simulink model "train_network"  (R2019a)
settings: Solver=VariableStepAuto  StartTime=0.0  StopTime=2400  RelTol=1e-3
values from neighbouring files (symbols this model uses):
  door_opening = [15 15 15 15 15 15 15]    [get_parameters.m]
  train_frequencies = struct    [get_parameters.m]
  travel_times = [ 0       60    0      0      0     0        0 ... (first row only)    [get_parameters.m]
undefined symbols (not defined in the file or in its folder): m, n
(part 2 of 2)

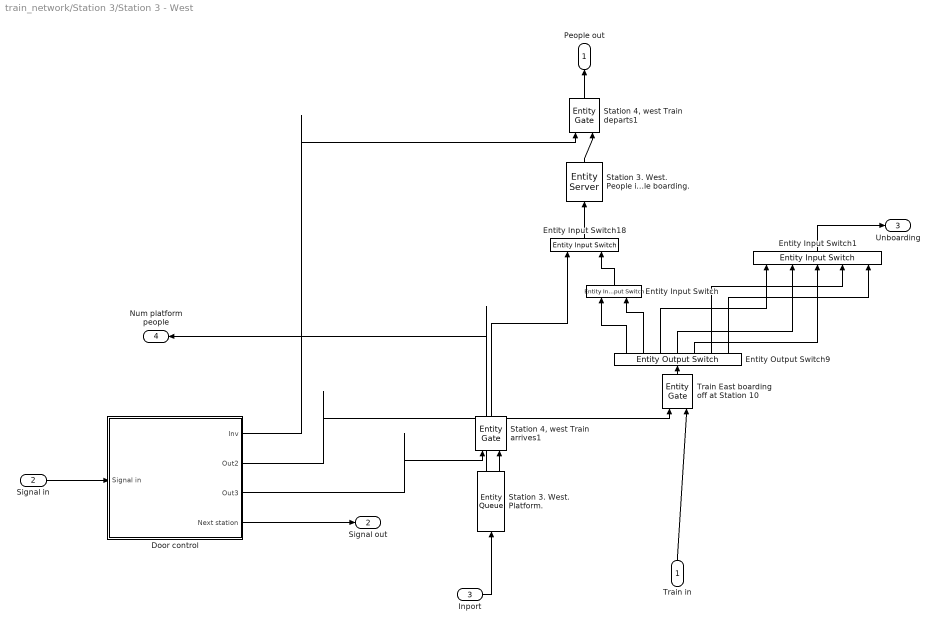
== system train_network/Station 3/Station 3 - West ==
  Train in : Inport
  Signal in : Inport  Port=2
  Inport : Inport  Port=3
  Door control : Subsystem
  Entity Input Switch : EntityInputSwitch  InputPortMessageModes=m,m  OutputPortMessageModes=m
  Entity Input Switch1 : EntityInputSwitch  InputPortMessageModes=m,m,m,m,m  OutputPortMessageModes=m  NumberInputPorts=5
      settings: InputPortMap=u1,u2,u3,u4,u5
  Entity Input Switch18 : EntityInputSwitch  InputPortMessageModes=m,m  OutputPortMessageModes=m
  Entity Output Switch9 : EntityOutputSwitch  InputPortMessageModes=m  OutputPortMessageModes=m,m,m,m,m,m,m  NumberOutputPorts=7  SwitchingCriterion=From attribute  SwitchAttributeName=EndStation
      settings: OutputPortMap=o0,o1,o2,o3,o4,o5,o6
  Station 3. West. People in train while boarding. : EntityServer  InputPortMessageModes=m  OutputPortMessageModes=m  Capacity=train_cap  ServiceTimeValue=0
  Station 3. West. Platform. : EntityQueue  InputPortMessageModes=m  OutputPortMessageModes=n,m  Capacity=inf  NumberEntitiesInBlock=on
      settings: OutputPortMap=o1,o5
  "Station 4, west Train departs1" : EntityGate  InputPortMessageModes=m,m  OutputPortMessageModes=m
  "Station 4, west Train arrives1" : EntityGate  InputPortMessageModes=m,m  OutputPortMessageModes=m
  Train East boarding off at Station 10 : EntityGate  InputPortMessageModes=m,m  OutputPortMessageModes=m
  People out : Outport
  Signal out : Outport  Port=2
  Unboarding : Outport  Port=3
  Num platform people : Outport  Port=4
  wires:
  Inport/1 -> Station 3. West. Platform./1
  Entity Input Switch18/1 -> Station 3. West. People in train while boarding./1
  Station 3. West. People in train while boarding./1 -> "Station 4, west Train departs1"/2
  Train in/1 -> Train East boarding off at Station 10/2
  "Station 4, west Train departs1"/1 -> People out/1
  Station 3. West. Platform./2 -> "Station 4, west Train arrives1"/2
  "Station 4, west Train arrives1"/1 -> Entity Input Switch18/1
  Door control/1(Inv) -> "Station 4, west Train departs1"/1
  Signal in/1 -> Door control/1(Signal in)
  Door control/4(Next station) -> Signal out/1
  Door control/2(Out2) -> Train East boarding off at Station 10/1
  Door control/3(Out3) -> "Station 4, west Train arrives1"/1
  Train East boarding off at Station 10/1 -> Entity Output Switch9/1
  Entity Input Switch/1 -> Entity Input Switch18/2
  Entity Output Switch9/1 -> Entity Input Switch/1
  Entity Output Switch9/2 -> Entity Input Switch/2
  Entity Input Switch1/1 -> Unboarding/1
  Entity Output Switch9/3 -> Entity Input Switch1/1
  Entity Output Switch9/4 -> Entity Input Switch1/2
  Entity Output Switch9/5 -> Entity Input Switch1/3
  Entity Output Switch9/6 -> Entity Input Switch1/4
  Entity Output Switch9/7 -> Entity Input Switch1/5
  Station 3. West. Platform./1 -> Num platform people/1

== system train_network/Station 3/Station 3 arrival ==
  Change their mind to depart at station 3. : EntityTerminator  InputPortMessageModes=m
  East.1 : EntityInputSwitch  InputPortMessageModes=m,m  OutputPortMessageModes=m
  Entity Output Switch3 : EntityOutputSwitch  InputPortMessageModes=m  OutputPortMessageModes=m,m,m,m,m,m,m  NumberOutputPorts=7  SwitchingCriterion=From attribute  SwitchAttributeName=EndStation
      settings: OutputPortMap=o0,o1,o2,o3,o4,o5,o6
  People arriving to station 1 : EntityGenerator  OutputPortMessageModes=m  TimeSource=MATLAB action  IntergenerationTimeAction=|  GenerateAction=|  AttributeName=EndStation|Timer|StartStation  AttributeInitialValue=0|1|3  EntityType=Structured  EntityTypeName=Inbound
      IntergenerationTimeAction=|
      | persistent rngInit;
      | if isempty(rngInit)
      |     seed = 173499;
      |     rng(seed);
      |     rngInit = true;
      | end
      | 
      | % Pattern: Exponential distribution
      | mu = lambda(3);
      | dt = -mu * log(1 - rand());
      GenerateAction=|
      | persistent rngInit;
      | if isempty(rngInit)
      |     seed = 12345;
      |     rng(seed);
      |     rngInit = true;
      | end
      | 
      | % Pattern: Arbitrary discrete distribution
      | % V: Value vector
      | % P: Probability vector
      | V = [1 2 3 4 5 6 7];
      | Ps = P(entity.StartStation,:);
      | entity.EndStation = randsample(V, 1, true, Ps);
      | 
      | coder.extrinsic("get_param");
      | entity.Timer = get_param("train_network", "SimulationTime");
  West.1 : EntityInputSwitch  InputPortMessageModes=m,m  OutputPortMessageModes=m
  North : Outport
  West : Outport  Port=2
  East : Outport  Port=3
  South : Outport  Port=4
  wires:
  Entity Output Switch3/1 -> West.1/1
  Entity Output Switch3/2 -> West.1/2
  West.1/1 -> West/1
  East.1/1 -> East/1
  Entity Output Switch3/7 -> South/1
  Entity Output Switch3/6 -> North/1
  Entity Output Switch3/3 -> Change their mind to depart at station 3./1
  People arriving to station 1/1 -> Entity Output Switch3/1
  Entity Output Switch3/4 -> East.1/1
  Entity Output Switch3/5 -> East.1/2

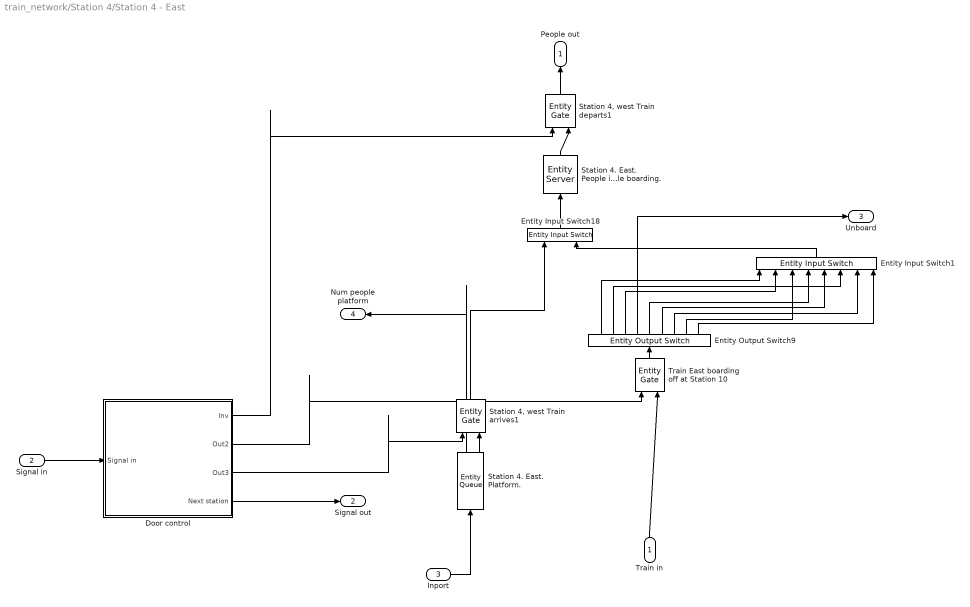
== system train_network/Station 4/Station 4 - East ==
  Train in : Inport
  Signal in : Inport  Port=2
  Inport : Inport  Port=3
  Door control : Subsystem
  Entity Input Switch1 : EntityInputSwitch  InputPortMessageModes=m,m,m,m,m,m,m,m  OutputPortMessageModes=m  NumberInputPorts=8
      settings: InputPortMap=u1,u2,u3,u4,u5,u6,u7,u8
  Entity Input Switch18 : EntityInputSwitch  InputPortMessageModes=m,m  OutputPortMessageModes=m
  Entity Output Switch9 : EntityOutputSwitch  InputPortMessageModes=m  OutputPortMessageModes=m,m,m,m,m,m,m,m,m  NumberOutputPorts=9  SwitchingCriterion=From attribute  SwitchAttributeName=EndStation
      settings: OutputPortMap=o0,o1,o2,o3,o4,o5,o6,o7,o8
  "Station 4, west Train departs1" : EntityGate  InputPortMessageModes=m,m  OutputPortMessageModes=m
  "Station 4, west Train arrives1" : EntityGate  InputPortMessageModes=m,m  OutputPortMessageModes=m
  Station 4. East. People in train while boarding. : EntityServer  InputPortMessageModes=m  OutputPortMessageModes=m  Capacity=train_cap  ServiceTimeValue=0
  Station 4. East. Platform. : EntityQueue  InputPortMessageModes=m  OutputPortMessageModes=n,m  Capacity=inf  NumberEntitiesInBlock=on
      settings: OutputPortMap=o1,o5
  Train East boarding off at Station 10 : EntityGate  InputPortMessageModes=m,m  OutputPortMessageModes=m
  People out : Outport
  Signal out : Outport  Port=2
  Unboard : Outport  Port=3
  Num people platform : Outport  Port=4
  wires:
  Inport/1 -> Station 4. East. Platform./1
  Entity Input Switch18/1 -> Station 4. East. People in train while boarding./1
  Station 4. East. People in train while boarding./1 -> "Station 4, west Train departs1"/2
  Train in/1 -> Train East boarding off at Station 10/2
  "Station 4, west Train departs1"/1 -> People out/1
  Station 4. East. Platform./2 -> "Station 4, west Train arrives1"/2
  "Station 4, west Train arrives1"/1 -> Entity Input Switch18/1
  Door control/1(Inv) -> "Station 4, west Train departs1"/1
  Signal in/1 -> Door control/1(Signal in)
  Door control/4(Next station) -> Signal out/1
  Door control/2(Out2) -> Train East boarding off at Station 10/1
  Door control/3(Out3) -> "Station 4, west Train arrives1"/1
  Entity Output Switch9/1 -> Entity Input Switch1/1
  Entity Output Switch9/2 -> Entity Input Switch1/6
  Entity Output Switch9/6 -> Entity Input Switch1/5
  Entity Output Switch9/3 -> Entity Input Switch1/2
  Entity Output Switch9/8 -> Entity Input Switch1/3
  Entity Output Switch9/5 -> Entity Input Switch1/4
  Entity Input Switch1/1 -> Entity Input Switch18/2
  Entity Output Switch9/4 -> Unboard/1
  Entity Output Switch9/7 -> Entity Input Switch1/7
  Entity Output Switch9/9 -> Entity Input Switch1/8
  Train East boarding off at Station 10/1 -> Entity Output Switch9/1
  Station 4. East. Platform./1 -> Num people platform/1

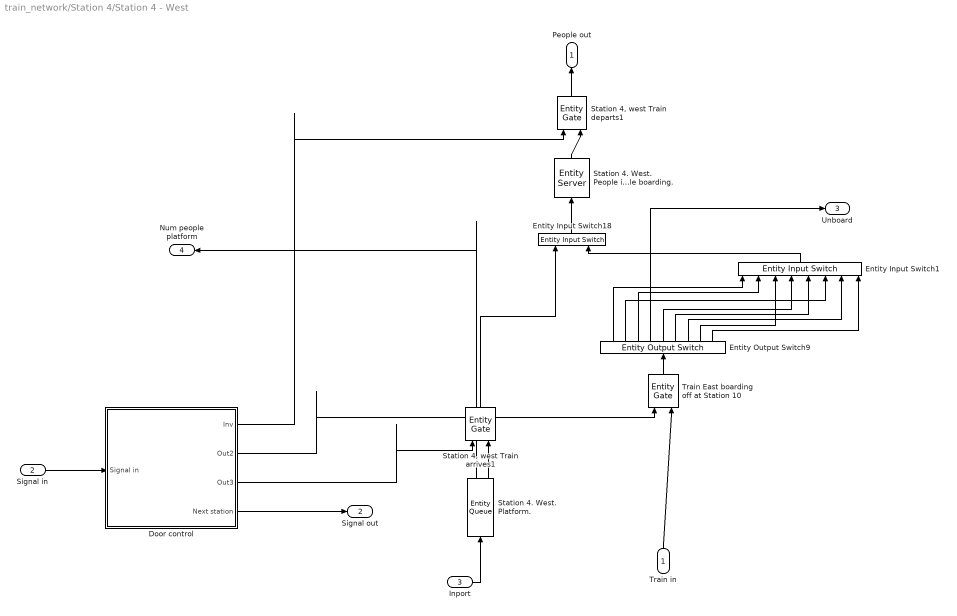
== system train_network/Station 4/Station 4 - West ==
  Train in : Inport
  Signal in : Inport  Port=2
  Inport : Inport  Port=3
  Door control : Subsystem
  Entity Input Switch1 : EntityInputSwitch  InputPortMessageModes=m,m,m,m,m,m,m,m  OutputPortMessageModes=m  NumberInputPorts=8
      settings: InputPortMap=u1,u2,u3,u4,u5,u6,u7,u8
  Entity Input Switch18 : EntityInputSwitch  InputPortMessageModes=m,m  OutputPortMessageModes=m
  Entity Output Switch9 : EntityOutputSwitch  InputPortMessageModes=m  OutputPortMessageModes=m,m,m,m,m,m,m,m,m  NumberOutputPorts=9  SwitchingCriterion=From attribute  SwitchAttributeName=EndStation
      settings: OutputPortMap=o0,o1,o2,o3,o4,o5,o6,o7,o8
  "Station 4, west Train departs1" : EntityGate  InputPortMessageModes=m,m  OutputPortMessageModes=m
  "Station 4, west Train arrives1" : EntityGate  InputPortMessageModes=m,m  OutputPortMessageModes=m
  Station 4. West. People in train while boarding. : EntityServer  InputPortMessageModes=m  OutputPortMessageModes=m  Capacity=train_cap  ServiceTimeValue=0
  Station 4. West. Platform. : EntityQueue  InputPortMessageModes=m  OutputPortMessageModes=n,m  Capacity=inf  NumberEntitiesInBlock=on
      settings: OutputPortMap=o1,o5
  Train East boarding off at Station 10 : EntityGate  InputPortMessageModes=m,m  OutputPortMessageModes=m
  People out : Outport
  Signal out : Outport  Port=2
  Unboard : Outport  Port=3
  Num people platform : Outport  Port=4
  wires:
  Inport/1 -> Station 4. West. Platform./1
  Entity Input Switch18/1 -> Station 4. West. People in train while boarding./1
  Station 4. West. People in train while boarding./1 -> "Station 4, west Train departs1"/2
  Train in/1 -> Train East boarding off at Station 10/2
  "Station 4, west Train departs1"/1 -> People out/1
  Station 4. West. Platform./2 -> "Station 4, west Train arrives1"/2
  "Station 4, west Train arrives1"/1 -> Entity Input Switch18/1
  Door control/1(Inv) -> "Station 4, west Train departs1"/1
  Signal in/1 -> Door control/1(Signal in)
  Door control/4(Next station) -> Signal out/1
  Door control/2(Out2) -> Train East boarding off at Station 10/1
  Door control/3(Out3) -> "Station 4, west Train arrives1"/1
  Entity Output Switch9/5 -> Entity Input Switch1/4
  Entity Input Switch1/1 -> Entity Input Switch18/2
  Entity Output Switch9/7 -> Entity Input Switch1/7
  Entity Output Switch9/9 -> Entity Input Switch1/8
  Entity Output Switch9/6 -> Entity Input Switch1/5
  Entity Output Switch9/8 -> Entity Input Switch1/3
  Entity Output Switch9/3 -> Entity Input Switch1/2
  Entity Output Switch9/2 -> Entity Input Switch1/6
  Entity Output Switch9/1 -> Entity Input Switch1/1
  Entity Output Switch9/4 -> Unboard/1
  Train East boarding off at Station 10/1 -> Entity Output Switch9/1
  Station 4. West. Platform./1 -> Num people platform/1

== system train_network/Station 5/Station 5 - East ==
  Train in : Inport
  Door control : Inport  Port=2
  " " : EntityGate  InputPortMessageModes=m,m  OutputPortMessageModes=m
  "Unboard " : Outport
  wires:
  " "/1 -> "Unboard "/1
  Door control/1 -> " "/1
  Train in/1 -> " "/2

== system train_network/Station 5/Station 5 - West ==
  Inport : Inport
  Departure blocking : EntityGate  InputPortMessageModes=m,m  OutputPortMessageModes=m
  Door controller : Subsystem
  "Station 5, west Train arrives1" : EntityGate  InputPortMessageModes=m,m  OutputPortMessageModes=m
  Station 5. West. People in train while boarding. : EntityServer  InputPortMessageModes=m  OutputPortMessageModes=m  Capacity=train_cap  ServiceTimeValue=0
  Station 5. West. Platform. : EntityQueue  InputPortMessageModes=m  OutputPortMessageModes=n,m  Capacity=inf  NumberEntitiesInBlock=on
      settings: OutputPortMap=o1,o5
  Train : Outport
  Signal : Outport  Port=2
  Platform number people : Outport  Port=3
  wires:
  Station 5. West. Platform./2 -> "Station 5, west Train arrives1"/2
  "Station 5, west Train arrives1"/1 -> Station 5. West. People in train while boarding./1
  Station 5. West. People in train while boarding./1 -> Departure blocking/2
  Departure blocking/1 -> Train/1
  Door controller/1(Next station) -> Signal/1
  Door controller/2(Departure) -> Departure blocking/1
  Door controller/3(Train door) -> "Station 5, west Train arrives1"/1
  Inport/1 -> Station 5. West. Platform./1
  Station 5. West. Platform./1 -> Platform number people/1

== system train_network/Station 6/Station 6 - North ==
  Train in : Inport
  Door control : Inport  Port=2
  " " : EntityGate  InputPortMessageModes=m,m  OutputPortMessageModes=m
  Unboard : Outport
  wires:
  Door control/1 -> " "/1
  Train in/1 -> " "/2
  " "/1 -> Unboard/1

== system train_network/Station 6/Station 6 - South ==
  Inport : Inport
  Departure blocking : EntityGate  InputPortMessageModes=m,m  OutputPortMessageModes=m
  Door controller : Subsystem
  "Station 5, west Train arrives1" : EntityGate  InputPortMessageModes=m,m  OutputPortMessageModes=m
  Station 6. South. People in train while boarding. : EntityServer  InputPortMessageModes=m  OutputPortMessageModes=m  Capacity=train_cap  ServiceTimeValue=0
  Station 6. South. Platform. : EntityQueue  InputPortMessageModes=m  OutputPortMessageModes=n,m  Capacity=inf  NumberEntitiesInBlock=on
      settings: OutputPortMap=o1,o5
  Train : Outport
  Signal : Outport  Port=2
  "People on platform " : Outport  Port=3
  wires:
  Station 6. South. Platform./2 -> "Station 5, west Train arrives1"/2
  "Station 5, west Train arrives1"/1 -> Station 6. South. People in train while boarding./1
  Station 6. South. People in train while boarding./1 -> Departure blocking/2
  Departure blocking/1 -> Train/1
  Door controller/1(Next station) -> Signal/1
  Door controller/2(Departure) -> Departure blocking/1
  Door controller/3(Train door) -> "Station 5, west Train arrives1"/1
  Inport/1 -> Station 6. South. Platform./1
  Station 6. South. Platform./1 -> "People on platform "/1

== system train_network/Station 7 /Station 7 - North ==
  Inport : Inport
  Departure blocking : EntityGate  InputPortMessageModes=m,m  OutputPortMessageModes=m
  Door controller : Subsystem
  "Station 7, north Train arrives1" : EntityGate  InputPortMessageModes=m,m  OutputPortMessageModes=m
  Station 7. North. People in train while boarding. : EntityServer  InputPortMessageModes=m  OutputPortMessageModes=m  Capacity=train_cap  ServiceTimeValue=0
  Station 7. North. Platform. : EntityQueue  InputPortMessageModes=m  OutputPortMessageModes=n,m  Capacity=inf  NumberEntitiesInBlock=on
      settings: OutputPortMap=o1,o5
  Train : Outport
  Signal : Outport  Port=2
  "Num people platform " : Outport  Port=3
  wires:
  Station 7. North. Platform./2 -> "Station 7, north Train arrives1"/2
  "Station 7, north Train arrives1"/1 -> Station 7. North. People in train while boarding./1
  Station 7. North. People in train while boarding./1 -> Departure blocking/2
  Departure blocking/1 -> Train/1
  Door controller/1(Next station) -> Signal/1
  Door controller/2(Departure) -> Departure blocking/1
  Door controller/3(Train door) -> "Station 7, north Train arrives1"/1
  Inport/1 -> Station 7. North. Platform./1
  Station 7. North. Platform./1 -> "Num people platform "/1

== system train_network/Station 7 /Station 7 - South ==
  Train in : Inport
  Door control : Inport  Port=2
  " " : EntityGate  InputPortMessageModes=m,m  OutputPortMessageModes=m
  Out1 : Outport
  wires:
  Door control/1 -> " "/1
  Train in/1 -> " "/2
  " "/1 -> Out1/1

== system train_network/Station 1/Station 1 - East/Door controller ==
  Delay : EntityServer  InputPortMessageModes=n,m  OutputPortMessageModes=m  Capacity=inf  ServiceTimeSource=Signal port  ServiceTimeValue=0
      settings: InputPortMap=u0,u2
  Delay offset : EntityServer  InputPortMessageModes=m  OutputPortMessageModes=m  Capacity=inf  ServiceTimeValue=train_offsets.E
  Door open time : Constant  Value=door_opening(1)
  Door signal : EntityGenerator  OutputPortMessageModes=m  TimeSource=Signal port  Period=300  GenerateEntityAtSimulationStart=off  AttributeName=entity  EntityTypeName=Entity  DataInitialValue=1
      settings: InputPortMap=u1
  Entity Input Switch17 : EntityInputSwitch  InputPortMessageModes=m,m  OutputPortMessageModes=m
  Entity Replicator2 : EntityReplicator  InputPortMessageModes=m  OutputPortMessageModes=m,m,m  NumberReplicas=2
      settings: OutputPortMap=o0,o1,o2
  Entity Replicator26 : EntityReplicator  InputPortMessageModes=m  OutputPortMessageModes=m,m
  Invert+delay : EntityServer  InputPortMessageModes=n,m  OutputPortMessageModes=m  Capacity=inf  ServiceTimeSource=Signal port  ServiceTimeValue=15  EntryAction=entity = -entity;
      settings: InputPortMap=u0,u2
  Inverter : EntityServer  InputPortMessageModes=m  OutputPortMessageModes=m  Capacity=inf  ServiceTimeValue=0  EntryAction=entity = -entity;
  Train frequency : Constant  Value=train_frequencies.E
  Next station : Outport
  Departure : Outport  Port=2
  Train door : Outport  Port=3
  wires:
  Door open time/1 -> Delay/1, Invert+delay/1
  Train frequency/1 -> Door signal/1
  Inverter/1 -> Departure/1
  Delay/1 -> Next station/1
  Invert+delay/1 -> Entity Input Switch17/1
  Entity Input Switch17/1 -> Entity Replicator26/1
  Entity Replicator26/1 -> Inverter/1
  Entity Replicator26/2 -> Train door/1
  Entity Replicator2/2 -> Entity Input Switch17/2
  Entity Replicator2/3 -> Delay/2
  Entity Replicator2/1 -> Invert+delay/2
  Door signal/1 -> Delay offset/1
  Delay offset/1 -> Entity Replicator2/1

== system train_network/Station 2/Station 2 - East/Door control ==
  Signal in : Inport
  Delay : EntityServer  InputPortMessageModes=n,m  OutputPortMessageModes=m  Capacity=inf  ServiceTimeSource=Signal port  ServiceTimeValue=0
      settings: InputPortMap=u0,u2
  Door open time : Constant  Value=door_opening(2)
  Entity Input Switch17 : EntityInputSwitch  InputPortMessageModes=m,m  OutputPortMessageModes=m
  Entity Replicator2 : EntityReplicator  InputPortMessageModes=m  OutputPortMessageModes=m,m,m  NumberReplicas=2
      settings: OutputPortMap=o0,o1,o2
  Entity Replicator26 : EntityReplicator  InputPortMessageModes=m  OutputPortMessageModes=m,m,m  NumberReplicas=2
      settings: OutputPortMap=o0,o1,o2
  Invert+delay : EntityServer  InputPortMessageModes=n,m  OutputPortMessageModes=m  Capacity=inf  ServiceTimeSource=Signal port  ServiceTimeValue=15  EntryAction=entity = -entity;
      settings: InputPortMap=u0,u2
  Inverter : EntityServer  InputPortMessageModes=m  OutputPortMessageModes=m  Capacity=inf  ServiceTimeValue=0  EntryAction=entity = -entity;
  Inv : Outport
  Out2 : Outport  Port=2
  Out3 : Outport  Port=3
  Next station : Outport  Port=4
  wires:
  Signal in/1 -> Entity Replicator2/1
  Entity Replicator2/3 -> Delay/2
  Delay/1 -> Next station/1
  Entity Replicator26/2 -> Out2/1
  Entity Replicator26/1 -> Inverter/1
  Door open time/1 -> Delay/1, Invert+delay/1
  Entity Replicator2/2 -> Entity Input Switch17/2
  Invert+delay/1 -> Entity Input Switch17/1
  Entity Replicator2/1 -> Invert+delay/2
  Entity Input Switch17/1 -> Entity Replicator26/1
  Entity Replicator26/3 -> Out3/1
  Inverter/1 -> Inv/1

== system train_network/Station 2/Station 2 - West/Door control ==
  Signal in : Inport
  Delay : EntityServer  InputPortMessageModes=n,m  OutputPortMessageModes=m  Capacity=inf  ServiceTimeSource=Signal port  ServiceTimeValue=0
      settings: InputPortMap=u0,u2
  Door open time : Constant  Value=door_opening(2)
  Entity Input Switch17 : EntityInputSwitch  InputPortMessageModes=m,m  OutputPortMessageModes=m
  Entity Replicator2 : EntityReplicator  InputPortMessageModes=m  OutputPortMessageModes=m,m,m  NumberReplicas=2
      settings: OutputPortMap=o0,o1,o2
  Entity Replicator26 : EntityReplicator  InputPortMessageModes=m  OutputPortMessageModes=m,m,m  NumberReplicas=2
      settings: OutputPortMap=o0,o1,o2
  Invert+delay : EntityServer  InputPortMessageModes=n,m  OutputPortMessageModes=m  Capacity=inf  ServiceTimeSource=Signal port  ServiceTimeValue=15  EntryAction=entity = -entity;
      settings: InputPortMap=u0,u2
  Inverter : EntityServer  InputPortMessageModes=m  OutputPortMessageModes=m  Capacity=inf  ServiceTimeValue=0  EntryAction=entity = -entity;
  Inv : Outport
  Out2 : Outport  Port=2
  Out3 : Outport  Port=3
  Next station : Outport  Port=4
  wires:
  Signal in/1 -> Entity Replicator2/1
  Entity Replicator2/3 -> Delay/2
  Delay/1 -> Next station/1
  Entity Replicator26/2 -> Out2/1
  Entity Replicator26/1 -> Inverter/1
  Door open time/1 -> Delay/1, Invert+delay/1
  Entity Replicator2/2 -> Entity Input Switch17/2
  Invert+delay/1 -> Entity Input Switch17/1
  Entity Replicator2/1 -> Invert+delay/2
  Entity Input Switch17/1 -> Entity Replicator26/1
  Entity Replicator26/3 -> Out3/1
  Inverter/1 -> Inv/1

== system train_network/Station 3/Station 3 - East/Door control ==
  Signal in : Inport
  Delay : EntityServer  InputPortMessageModes=n,m  OutputPortMessageModes=m  Capacity=inf  ServiceTimeSource=Signal port  ServiceTimeValue=0
      settings: InputPortMap=u0,u2
  Door open time : Constant  Value=door_opening(3)
  Entity Input Switch17 : EntityInputSwitch  InputPortMessageModes=m,m  OutputPortMessageModes=m
  Entity Replicator2 : EntityReplicator  InputPortMessageModes=m  OutputPortMessageModes=m,m,m  NumberReplicas=2
      settings: OutputPortMap=o0,o1,o2
  Entity Replicator26 : EntityReplicator  InputPortMessageModes=m  OutputPortMessageModes=m,m,m  NumberReplicas=2
      settings: OutputPortMap=o0,o1,o2
  Invert+delay : EntityServer  InputPortMessageModes=n,m  OutputPortMessageModes=m  Capacity=inf  ServiceTimeSource=Signal port  ServiceTimeValue=15  EntryAction=entity = -entity;
      settings: InputPortMap=u0,u2
  Inverter : EntityServer  InputPortMessageModes=m  OutputPortMessageModes=m  Capacity=inf  ServiceTimeValue=0  EntryAction=entity = -entity;
  Inv : Outport
  Out2 : Outport  Port=2
  Out3 : Outport  Port=3
  Next station : Outport  Port=4
  wires:
  Signal in/1 -> Entity Replicator2/1
  Entity Replicator2/3 -> Delay/2
  Delay/1 -> Next station/1
  Entity Replicator2/2 -> Entity Input Switch17/2
  Entity Replicator26/2 -> Out2/1
  Entity Replicator26/1 -> Inverter/1
  Door open time/1 -> Delay/1, Invert+delay/1
  Invert+delay/1 -> Entity Input Switch17/1
  Entity Replicator2/1 -> Invert+delay/2
  Entity Input Switch17/1 -> Entity Replicator26/1
  Entity Replicator26/3 -> Out3/1
  Inverter/1 -> Inv/1

== system train_network/Station 3/Station 3 - North/Door control ==
  Signal in : Inport
  Delay : EntityServer  InputPortMessageModes=n,m  OutputPortMessageModes=m  Capacity=inf  ServiceTimeSource=Signal port  ServiceTimeValue=0
      settings: InputPortMap=u0,u2
  Door open time : Constant  Value=door_opening(3)
  Entity Input Switch17 : EntityInputSwitch  InputPortMessageModes=m,m  OutputPortMessageModes=m
  Entity Replicator2 : EntityReplicator  InputPortMessageModes=m  OutputPortMessageModes=m,m,m  NumberReplicas=2
      settings: OutputPortMap=o0,o1,o2
  Entity Replicator26 : EntityReplicator  InputPortMessageModes=m  OutputPortMessageModes=m,m,m  NumberReplicas=2
      settings: OutputPortMap=o0,o1,o2
  Invert+delay : EntityServer  InputPortMessageModes=n,m  OutputPortMessageModes=m  Capacity=inf  ServiceTimeSource=Signal port  ServiceTimeValue=15  EntryAction=entity = -entity;
      settings: InputPortMap=u0,u2
  Inverter : EntityServer  InputPortMessageModes=m  OutputPortMessageModes=m  Capacity=inf  ServiceTimeValue=0  EntryAction=entity = -entity;
  Inv : Outport
  Out2 : Outport  Port=2
  Out3 : Outport  Port=3
  Next station : Outport  Port=4
  wires:
  Signal in/1 -> Entity Replicator2/1
  Entity Replicator2/3 -> Delay/2
  Delay/1 -> Next station/1
  Entity Replicator26/2 -> Out2/1
  Entity Replicator26/1 -> Inverter/1
  Door open time/1 -> Delay/1, Invert+delay/1
  Entity Replicator2/2 -> Entity Input Switch17/2
  Invert+delay/1 -> Entity Input Switch17/1
  Entity Replicator2/1 -> Invert+delay/2
  Entity Input Switch17/1 -> Entity Replicator26/1
  Entity Replicator26/3 -> Out3/1
  Inverter/1 -> Inv/1

== system train_network/Station 3/Station 3 - South/Door control ==
  Signal in : Inport
  Delay : EntityServer  InputPortMessageModes=n,m  OutputPortMessageModes=m  Capacity=inf  ServiceTimeSource=Signal port  ServiceTimeValue=0
      settings: InputPortMap=u0,u2
  Door open time : Constant  Value=door_opening(3)
  Entity Input Switch17 : EntityInputSwitch  InputPortMessageModes=m,m  OutputPortMessageModes=m
  Entity Replicator2 : EntityReplicator  InputPortMessageModes=m  OutputPortMessageModes=m,m,m  NumberReplicas=2
      settings: OutputPortMap=o0,o1,o2
  Entity Replicator26 : EntityReplicator  InputPortMessageModes=m  OutputPortMessageModes=m,m,m  NumberReplicas=2
      settings: OutputPortMap=o0,o1,o2
  Invert+delay : EntityServer  InputPortMessageModes=n,m  OutputPortMessageModes=m  Capacity=inf  ServiceTimeSource=Signal port  ServiceTimeValue=15  EntryAction=entity = -entity;
      settings: InputPortMap=u0,u2
  Inverter : EntityServer  InputPortMessageModes=m  OutputPortMessageModes=m  Capacity=inf  ServiceTimeValue=0  EntryAction=entity = -entity;
  Inv : Outport
  Out2 : Outport  Port=2
  Out3 : Outport  Port=3
  Next station : Outport  Port=4
  wires:
  Signal in/1 -> Entity Replicator2/1
  Entity Replicator2/3 -> Delay/2
  Delay/1 -> Next station/1
  Entity Replicator26/2 -> Out2/1
  Entity Replicator26/1 -> Inverter/1
  Door open time/1 -> Delay/1, Invert+delay/1
  Entity Replicator2/2 -> Entity Input Switch17/2
  Invert+delay/1 -> Entity Input Switch17/1
  Entity Replicator2/1 -> Invert+delay/2
  Entity Input Switch17/1 -> Entity Replicator26/1
  Entity Replicator26/3 -> Out3/1
  Inverter/1 -> Inv/1

== system train_network/Station 3/Station 3 - West/Door control ==
  Signal in : Inport
  Delay : EntityServer  InputPortMessageModes=n,m  OutputPortMessageModes=m  Capacity=inf  ServiceTimeSource=Signal port  ServiceTimeValue=0
      settings: InputPortMap=u0,u2
  Door open time : Constant  Value=door_opening(3)
  Entity Input Switch17 : EntityInputSwitch  InputPortMessageModes=m,m  OutputPortMessageModes=m
  Entity Replicator2 : EntityReplicator  InputPortMessageModes=m  OutputPortMessageModes=m,m,m  NumberReplicas=2
      settings: OutputPortMap=o0,o1,o2
  Entity Replicator26 : EntityReplicator  InputPortMessageModes=m  OutputPortMessageModes=m,m,m  NumberReplicas=2
      settings: OutputPortMap=o0,o1,o2
  Invert+delay : EntityServer  InputPortMessageModes=n,m  OutputPortMessageModes=m  Capacity=inf  ServiceTimeSource=Signal port  ServiceTimeValue=15  EntryAction=entity = -entity;
      settings: InputPortMap=u0,u2
  Inverter : EntityServer  InputPortMessageModes=m  OutputPortMessageModes=m  Capacity=inf  ServiceTimeValue=0  EntryAction=entity = -entity;
  Inv : Outport
  Out2 : Outport  Port=2
  Out3 : Outport  Port=3
  Next station : Outport  Port=4
  wires:
  Signal in/1 -> Entity Replicator2/1
  Entity Replicator2/3 -> Delay/2
  Delay/1 -> Next station/1
  Entity Replicator26/2 -> Out2/1
  Entity Replicator26/1 -> Inverter/1
  Door open time/1 -> Delay/1, Invert+delay/1
  Entity Replicator2/2 -> Entity Input Switch17/2
  Invert+delay/1 -> Entity Input Switch17/1
  Entity Replicator2/1 -> Invert+delay/2
  Entity Input Switch17/1 -> Entity Replicator26/1
  Entity Replicator26/3 -> Out3/1
  Inverter/1 -> Inv/1

== system train_network/Station 4/Station 4 - East/Door control ==
  Signal in : Inport
  Delay : EntityServer  InputPortMessageModes=n,m  OutputPortMessageModes=m  Capacity=inf  ServiceTimeSource=Signal port  ServiceTimeValue=0
      settings: InputPortMap=u0,u2
  Door open time : Constant  Value=door_opening(4)
  Entity Input Switch17 : EntityInputSwitch  InputPortMessageModes=m,m  OutputPortMessageModes=m
  Entity Replicator2 : EntityReplicator  InputPortMessageModes=m  OutputPortMessageModes=m,m,m  NumberReplicas=2
      settings: OutputPortMap=o0,o1,o2
  Entity Replicator26 : EntityReplicator  InputPortMessageModes=m  OutputPortMessageModes=m,m,m  NumberReplicas=2
      settings: OutputPortMap=o0,o1,o2
  Invert+delay : EntityServer  InputPortMessageModes=n,m  OutputPortMessageModes=m  Capacity=inf  ServiceTimeSource=Signal port  ServiceTimeValue=15  EntryAction=entity = -entity;
      settings: InputPortMap=u0,u2
  Inverter : EntityServer  InputPortMessageModes=m  OutputPortMessageModes=m  Capacity=inf  ServiceTimeValue=0  EntryAction=entity = -entity;
  Inv : Outport
  Out2 : Outport  Port=2
  Out3 : Outport  Port=3
  Next station : Outport  Port=4
  wires:
  Signal in/1 -> Entity Replicator2/1
  Entity Replicator2/3 -> Delay/2
  Delay/1 -> Next station/1
  Entity Replicator26/2 -> Out2/1
  Entity Replicator26/1 -> Inverter/1
  Door open time/1 -> Delay/1, Invert+delay/1
  Entity Replicator2/2 -> Entity Input Switch17/2
  Invert+delay/1 -> Entity Input Switch17/1
  Entity Replicator2/1 -> Invert+delay/2
  Entity Input Switch17/1 -> Entity Replicator26/1
  Entity Replicator26/3 -> Out3/1
  Inverter/1 -> Inv/1

== system train_network/Station 4/Station 4 - West/Door control ==
  Signal in : Inport
  Delay : EntityServer  InputPortMessageModes=n,m  OutputPortMessageModes=m  Capacity=inf  ServiceTimeSource=Signal port  ServiceTimeValue=0
      settings: InputPortMap=u0,u2
  Door open time : Constant  Value=door_opening(4)
  Entity Input Switch17 : EntityInputSwitch  InputPortMessageModes=m,m  OutputPortMessageModes=m
  Entity Replicator2 : EntityReplicator  InputPortMessageModes=m  OutputPortMessageModes=m,m,m  NumberReplicas=2
      settings: OutputPortMap=o0,o1,o2
  Entity Replicator26 : EntityReplicator  InputPortMessageModes=m  OutputPortMessageModes=m,m,m  NumberReplicas=2
      settings: OutputPortMap=o0,o1,o2
  Invert+delay : EntityServer  InputPortMessageModes=n,m  OutputPortMessageModes=m  Capacity=inf  ServiceTimeSource=Signal port  ServiceTimeValue=15  EntryAction=entity = -entity;
      settings: InputPortMap=u0,u2
  Inverter : EntityServer  InputPortMessageModes=m  OutputPortMessageModes=m  Capacity=inf  ServiceTimeValue=0  EntryAction=entity = -entity;
  Inv : Outport
  Out2 : Outport  Port=2
  Out3 : Outport  Port=3
  Next station : Outport  Port=4
  wires:
  Signal in/1 -> Entity Replicator2/1
  Entity Replicator2/3 -> Delay/2
  Delay/1 -> Next station/1
  Entity Replicator26/2 -> Out2/1
  Entity Replicator26/1 -> Inverter/1
  Door open time/1 -> Delay/1, Invert+delay/1
  Entity Replicator2/2 -> Entity Input Switch17/2
  Invert+delay/1 -> Entity Input Switch17/1
  Entity Replicator2/1 -> Invert+delay/2
  Entity Input Switch17/1 -> Entity Replicator26/1
  Entity Replicator26/3 -> Out3/1
  Inverter/1 -> Inv/1

== system train_network/Station 5/Station 5 - West/Door controller ==
  Delay : EntityServer  InputPortMessageModes=n,m  OutputPortMessageModes=m  Capacity=inf  ServiceTimeSource=Signal port  ServiceTimeValue=0
      settings: InputPortMap=u0,u2
  Door open time : Constant  Value=door_opening(5)
  Door signal : EntityGenerator  OutputPortMessageModes=m  TimeSource=Signal port  Period=300  GenerateEntityAtSimulationStart=off  AttributeName=entity  EntityTypeName=Entity  DataInitialValue=1
      settings: InputPortMap=u1
  Entity Input Switch17 : EntityInputSwitch  InputPortMessageModes=m,m  OutputPortMessageModes=m
  Entity Replicator2 : EntityReplicator  InputPortMessageModes=m  OutputPortMessageModes=m,m,m  NumberReplicas=2
      settings: OutputPortMap=o0,o1,o2
  Entity Replicator26 : EntityReplicator  InputPortMessageModes=m  OutputPortMessageModes=m,m
  Entity Server : EntityServer  InputPortMessageModes=m  OutputPortMessageModes=m  Capacity=inf  ServiceTimeValue=train_offsets.W
  Invert+delay : EntityServer  InputPortMessageModes=n,m  OutputPortMessageModes=m  Capacity=inf  ServiceTimeSource=Signal port  ServiceTimeValue=15  EntryAction=entity = -entity;
      settings: InputPortMap=u0,u2
  Inverter : EntityServer  InputPortMessageModes=m  OutputPortMessageModes=m  Capacity=inf  ServiceTimeValue=0  EntryAction=entity = -entity;
  Train frequency : Constant  Value=train_frequencies.W
  Next station : Outport
  Departure : Outport  Port=2
  Train door : Outport  Port=3
  wires:
  Door open time/1 -> Delay/1, Invert+delay/1
  Train frequency/1 -> Door signal/1
  Inverter/1 -> Departure/1
  Delay/1 -> Next station/1
  Invert+delay/1 -> Entity Input Switch17/1
  Entity Input Switch17/1 -> Entity Replicator26/1
  Entity Replicator26/1 -> Inverter/1
  Entity Replicator26/2 -> Train door/1
  Entity Replicator2/2 -> Entity Input Switch17/2
  Entity Replicator2/3 -> Delay/2
  Entity Replicator2/1 -> Invert+delay/2
  Door signal/1 -> Entity Server/1
  Entity Server/1 -> Entity Replicator2/1

== system train_network/Station 6/Station 6 - South/Door controller ==
  Delay : EntityServer  InputPortMessageModes=n,m  OutputPortMessageModes=m  Capacity=inf  ServiceTimeSource=Signal port  ServiceTimeValue=0
      settings: InputPortMap=u0,u2
  Door open time : Constant  Value=door_opening(6)
  Door signal : EntityGenerator  OutputPortMessageModes=m  TimeSource=Signal port  Period=300  GenerateEntityAtSimulationStart=off  AttributeName=entity  EntityTypeName=Entity  DataInitialValue=1
      settings: InputPortMap=u1
  Entity Input Switch17 : EntityInputSwitch  InputPortMessageModes=m,m  OutputPortMessageModes=m
  Entity Replicator2 : EntityReplicator  InputPortMessageModes=m  OutputPortMessageModes=m,m,m  NumberReplicas=2
      settings: OutputPortMap=o0,o1,o2
  Entity Replicator26 : EntityReplicator  InputPortMessageModes=m  OutputPortMessageModes=m,m
  Entity Server : EntityServer  InputPortMessageModes=m  OutputPortMessageModes=m  Capacity=inf  ServiceTimeValue=train_offsets.S
  Invert+delay : EntityServer  InputPortMessageModes=n,m  OutputPortMessageModes=m  Capacity=inf  ServiceTimeSource=Signal port  ServiceTimeValue=15  EntryAction=entity = -entity;
      settings: InputPortMap=u0,u2
  Inverter : EntityServer  InputPortMessageModes=m  OutputPortMessageModes=m  Capacity=inf  ServiceTimeValue=0  EntryAction=entity = -entity;
  Train frequency : Constant  Value=train_frequencies.S
  Next station : Outport
  Departure : Outport  Port=2
  Train door : Outport  Port=3
  wires:
  Door open time/1 -> Delay/1, Invert+delay/1
  Train frequency/1 -> Door signal/1
  Inverter/1 -> Departure/1
  Delay/1 -> Next station/1
  Invert+delay/1 -> Entity Input Switch17/1
  Entity Input Switch17/1 -> Entity Replicator26/1
  Entity Replicator26/1 -> Inverter/1
  Entity Replicator26/2 -> Train door/1
  Entity Replicator2/2 -> Entity Input Switch17/2
  Entity Replicator2/3 -> Delay/2
  Entity Replicator2/1 -> Invert+delay/2
  Door signal/1 -> Entity Server/1
  Entity Server/1 -> Entity Replicator2/1

== system train_network/Station 7 /Station 7 - North/Door controller ==
  Delay : EntityServer  InputPortMessageModes=n,m  OutputPortMessageModes=m  Capacity=inf  ServiceTimeSource=Signal port  ServiceTimeValue=0
      settings: InputPortMap=u0,u2
  Door open time : Constant  Value=door_opening(7)
  Door signal : EntityGenerator  OutputPortMessageModes=m  TimeSource=Signal port  Period=300  GenerateEntityAtSimulationStart=off  AttributeName=entity  EntityTypeName=Entity  DataInitialValue=1
      settings: InputPortMap=u1
  Entity Input Switch17 : EntityInputSwitch  InputPortMessageModes=m,m  OutputPortMessageModes=m
  Entity Replicator2 : EntityReplicator  InputPortMessageModes=m  OutputPortMessageModes=m,m,m  NumberReplicas=2
      settings: OutputPortMap=o0,o1,o2
  Entity Replicator26 : EntityReplicator  InputPortMessageModes=m  OutputPortMessageModes=m,m
  Entity Server : EntityServer  InputPortMessageModes=m  OutputPortMessageModes=m  Capacity=inf  ServiceTimeValue=train_offsets.N
  Invert+delay : EntityServer  InputPortMessageModes=n,m  OutputPortMessageModes=m  Capacity=inf  ServiceTimeSource=Signal port  ServiceTimeValue=15  EntryAction=entity = -entity;
      settings: InputPortMap=u0,u2
  Inverter : EntityServer  InputPortMessageModes=m  OutputPortMessageModes=m  Capacity=inf  ServiceTimeValue=0  EntryAction=entity = -entity;
  Train frequency : Constant  Value=train_frequencies.N
  Next station : Outport
  Departure : Outport  Port=2
  Train door : Outport  Port=3
  wires:
  Door open time/1 -> Delay/1, Invert+delay/1
  Train frequency/1 -> Door signal/1
  Inverter/1 -> Departure/1
  Delay/1 -> Next station/1
  Invert+delay/1 -> Entity Input Switch17/1
  Entity Input Switch17/1 -> Entity Replicator26/1
  Entity Replicator26/1 -> Inverter/1
  Entity Replicator26/2 -> Train door/1
  Entity Replicator2/2 -> Entity Input Switch17/2
  Entity Replicator2/3 -> Delay/2
  Entity Replicator2/1 -> Invert+delay/2
  Door signal/1 -> Entity Server/1
  Entity Server/1 -> Entity Replicator2/1
